simulink model "simple_pendulum_1D"  (R2025b)
settings: Solver=ode45  StartTime=0.0  StopTime=10.0  MaxStep=0.01  RelTol=1e-3  EnableMultiTasking=on
settings Model: Creator=nike  LastModifiedBy=ZBook Fury
settings SolverCC: AlgebraicLoopSolver=TrustRegion
settings DataIOCC: LimitDataPoints=on  SaveFormat=Array  SignalLoggingSaveFormat=ModelDataLogs  ReturnWorkspaceOutputs=off
settings OptimizationCC: ExpressionDepthLimit=2147483647.0  LifeSpan=inf
settings DebuggingCC: UnderspecifiedInitializationDetection=Classic  MergeDetectMultiDrivingBlocksExec=none  SolverPrmCheckMsg=warning  FcnCallInpInsideContextMsg=warning  UnconnectedInputMsg=warning  UnconnectedOutputMsg=warning  UnconnectedLineMsg=warning  StateNameClashWarn=warning  SFUnexpectedBacktrackingDiag=warning  SFNoUnconditionalDefaultTransitionDiag=warning  SFExecutionAtInitializationDiag=none  ArithmeticOperatorsInVariantConditions=warning
settings HardwareCC: ProdBitPerPointer=32.0  ProdBitPerSizeT=32.0  ProdBitPerPtrDiffT=32.0  ProdLargestAtomicFloat=None  ProdIntDivRoundTo=Undefined  ProdEndianess=Unspecified  ProdWordSize=32.0  ProdHWDeviceType=32-bit Generic
settings ModelReferenceCC: PropagateSignalLabelsOutOfModel=off
settings SFSimCC: SimUseLocalCustomCode=off  CustomCodeUndefinedFunction=UseInterfaceOnly
settings RTWCC: RTWUseLocalCustomCode=off  GPUComputeCapability=3.5
settings CodeAppCC: StateflowObjectComments=on
settings GRTTargetCC: TargetLangStandard=C89/C90 (ANSI)  CombineOutputUpdateFcns=off  GRTInterface=on
settings ConfigComp: CovMetricSettings=dw  CovSaveCumulativeToWorkspaceVar=on  CovSaveSingleToWorkspaceVar=on  CovExternalEMLEnable=off

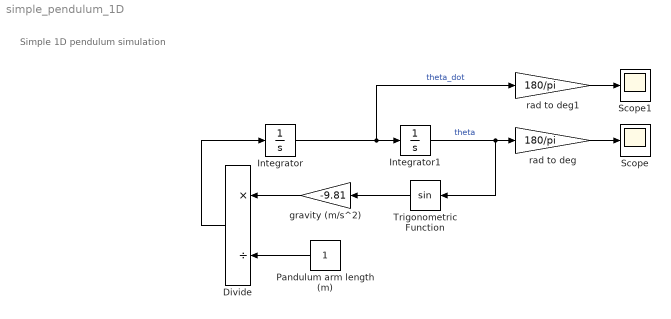
== system simple_pendulum_1D ==
  note: Simple 1D pendulum simulation
  Divide : Product  Inputs=*/
  Integrator : Integrator  InitialCondition=100*pi/180
  Integrator1 : Integrator  InitialCondition=pi/3
  Pandulum arm length (m) : Constant
  Scope : Scope
      settings: ActiveDisplayYMinimum=-87.291788227303783  ActiveDisplayYMaximum=87.288070005190491
  Scope1 : Scope
      settings: ActiveDisplayYMinimum=-224.31946732891808  ActiveDisplayYMaximum=224.31938749915366
  Trigonometric Function : Trigonometry
  gravity (m/s^2) : Gain  Gain=-9.81
  rad to deg : Gain  Gain=180/pi
  rad to deg1 : Gain  Gain=180/pi
  wires:
  Integrator/1 -> rad to deg1/1, Integrator1/1  "theta_dot"
  Integrator1/1 -> rad to deg/1, Trigonometric Function/1  "theta"
  Trigonometric Function/1 -> gravity (m/s^2)/1
  gravity (m/s^2)/1 -> Divide/1
  Divide/1 -> Integrator/1
  Pandulum arm length (m)/1 -> Divide/2
  rad to deg/1 -> Scope/1
  rad to deg1/1 -> Scope1/1
